simulink model "QPSK_send_new"  (Simulink 9.0)
settings: Solver=FixedStepDiscrete  StartTime=0.0  StopTime=inf  RelTol=1e-3
PreLoadFcn:
  | setenv('MW_MINGW64_LOC','C:\TDM-GCC-64')
  | load('qpsktxrx.mat')
StartFcn:
  | load('qpsktxrx.mat')
  | tic
StopFcn:
  | toc;
values from neighbouring files (symbols this model uses):
  data_send = [data_send frame]    [myimg_transfer.m]    (also in test_data.m = [data_send, head, data(i:i+20*9-1)]; test_data_v2.m = [data_send, frame])
  qpsktxrx =     [qpsktxrx.mat]
undefined symbols (not defined in the file or in its folder): CRC, gcbh, none, rcfiltgaincompat, videoinput
libraries: UN_HIL_Lib x2, commcrc2 x1, imaqlib x1, commutil2 x1, dspsigops x1, commsequence2 x1, commdigbbndpm3 x1, commfilt2 x1
Description:
  | QPSK Transmitter and Receiver.
  | 
  | This model shows the implementation of a QPSK transmitter and receiver.
settings Model: FPTRunName=Active  Creator=The MathWorks Inc.  LastModifiedBy=minel
settings DataIOCC: LimitDataPoints=on  SignalLoggingSaveFormat=ModelDataLogs  SaveOutput=off  SaveTime=off
settings OptimizationCC: BooleanDataType=off  DefaultParameterBehavior=Inlined  ExpressionDepthLimit=2147483647  LocalBlockOutputs=off
settings DebuggingCC: AlgebraicLoopMsg=error  SolverPrmCheckMsg=warning  SingleTaskRateTransMsg=error  ParameterPrecisionLossMsg=none  FcnCallInpInsideContextMsg=warning  StateNameClashWarn=warning
settings HardwareCC: TargetBitPerPointer=64  TargetBitPerSizeT=64  TargetBitPerPtrDiffT=64  TargetLongLongMode=on  TargetIntDivRoundTo=Zero  TargetEndianess=LittleEndian  TargetWordSize=64  TargetHWDeviceType=Generic->MATLAB Host Computer  ProdEqTarget=off
settings GRTTargetCC: GeneratePreprocessorConditionals=Disable all
settings ConfigComp: CovSFcnEnable=off
settings SimEventsCC: propDiagStatOutput=1  propPreventDuplicateEvents=0

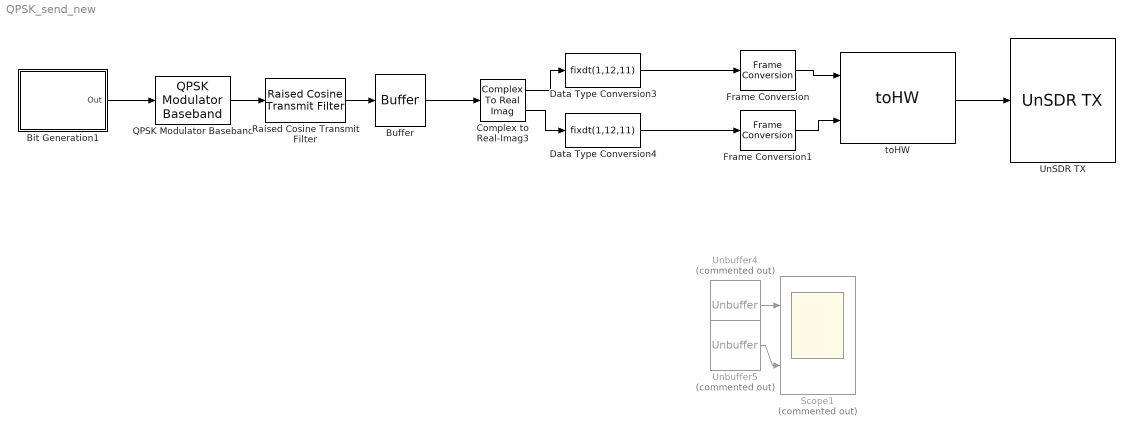
== system QPSK_send_new ==
  Bit Generation1 : Subsystem
      mask Display: disp('Bits Generation')
  Buffer : Buffer  N=4096  OutputFrames=off
  Complex to Real-Imag3 : ComplexToRealImag
  Data Type Conversion3 : DataTypeConversion  OutDataTypeStr=fixdt(1,12,11)
  Data Type Conversion4 : DataTypeConversion  OutDataTypeStr=fixdt(1,12,11)
  Frame Conversion : FrameConversion  InheritSamplingMode=off  OutFrame=Sample-based
  Frame Conversion1 : FrameConversion  InheritSamplingMode=off  OutFrame=Sample-based
  QPSK Modulator Baseband : commdigbbndpm3/QPSK Modulator Baseband  InType=Bit  Enc=Gray  Ph=pi/4  outDtype=double  outWordLen=16  outUDDataType=sfix(16)  outFracLenMode=Best precision  outFracLen=15  outDataTypeStr=double  outLastDataTypeStr=double
  Raised Cosine Transmit Filter : commfilt2/Raised Cosine Transmit Filter  filtType=Square root  R=0.5  filtSpan=2*((qpsktxrx.RaisedCosineFilterSpan)/2)  N=qpsktxrx.Upsampling  filterGain=rcfiltgaincompat(gcbh)  InputProcessing=Columns as channels (frame based)  RateOptions=Enforce single-rate processing  framing=Mute  checkCoeff=off  variableName=rcTxFilt  checkGain=Normalized  sampMode=Mute  saveAsFlag=0  currentFiltSpan=2*((qpsktxrx.RaisedCosineFilterSpan)/2)  D=(qpsktxrx.RaisedCosineFilterSpan)/2  launchFVT=off  roundingMode=Floor  overflowMode=off  coeffDataTypeStr=Inherit: Same word length as input  coeffMin=[]  coeffMax=[]  coeffLastDataTypeStr=Inherit: Same word length as input  outputDataTypeStr=Inherit: Same as accumulator  outputMin=[]  outputMax=[]  outputLastDataTypeStr=Inherit: Same as accumulator
  Scope1 : Scope  Commented=on  NumInputPorts=2
  UnSDR TX : UN_HIL_Lib/UnSDR TX  SystemSampleTime=-1
      settings: SourceProductName=HIL Blockset
  Unbuffer4 : Unbuffer  Commented=on
  Unbuffer5 : Unbuffer  Commented=on
  toHW : UN_HIL_Lib/toHW  SystemSampleTime=-1
      settings: SourceProductName=HIL Blockset
  wires:
  Unbuffer5/1 -> Scope1/2
  Unbuffer4/1 -> Scope1/1
  Data Type Conversion3/1 -> Frame Conversion/1
  Data Type Conversion4/1 -> Frame Conversion1/1
  Complex to Real-Imag3/2 -> Data Type Conversion4/1
  Complex to Real-Imag3/1 -> Data Type Conversion3/1
  Bit Generation1/1(Out) -> QPSK Modulator Baseband/1
  QPSK Modulator Baseband/1 -> Raised Cosine Transmit Filter/1
  toHW/1 -> UnSDR TX/1
  Frame Conversion/1 -> toHW/1
  Frame Conversion1/1 -> toHW/2
  Raised Cosine Transmit Filter/1 -> Buffer/1
  Buffer/1 -> Complex to Real-Imag3/1

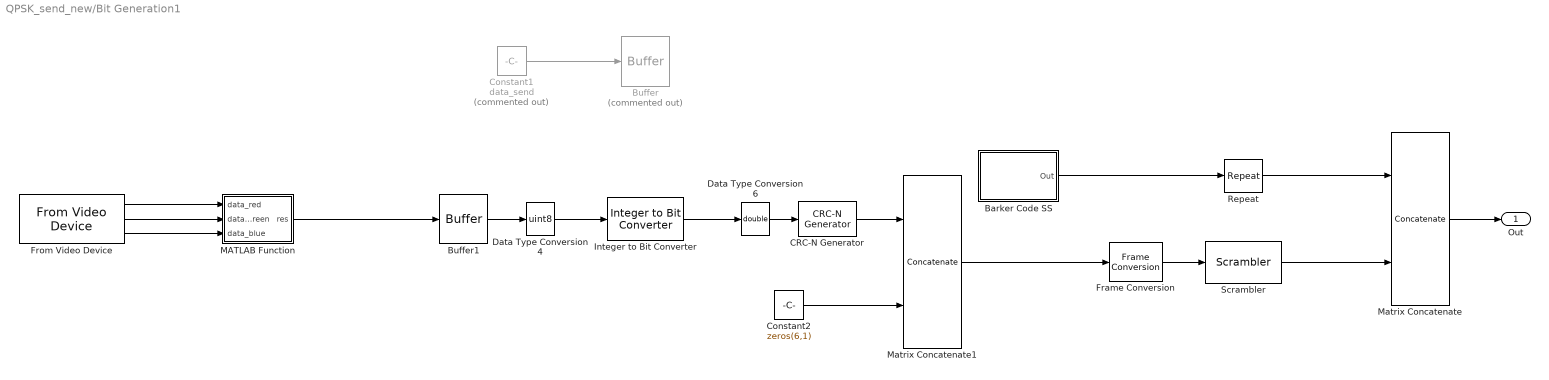
== system QPSK_send_new/Bit Generation1 ==
  Barker Code SS : Subsystem
      mask Display: disp('Unipolar\nBarker Code')
  Buffer : Buffer  Commented=on  N=20  OutputFrames=off
  Buffer1 : Buffer  N=20  OutputFrames=off
  CRC-N Generator : commcrc2/CRC-N Generator  crcMethod=CRC-8  iniStates=[0]  numChecksums=1
      settings: SourceProductName=Communications System Toolbox  SourceProductBaseCode=CM
  Constant1 : Constant  Commented=on  Value=data_send  SampleTime=1/2100/5*102470*5*5250*4096/1e8
  Constant2 : Constant  Value=zeros(6,1)  VectorParams1D=off  SampleTime=-1
  Data Type Conversion4 : DataTypeConversion  OutDataTypeStr=uint8
  Data Type Conversion6 : DataTypeConversion  OutDataTypeStr=double
  Frame Conversion : FrameConversion  InheritSamplingMode=off  OutFrame=Sample-based
  From Video Device : imaqlib/From Video Device  DeviceMenu=winvideo 1 (Integrated Webcam)  Device=winvideo 1 (Integrated Webcam)  ObjConstructor=videoinput('winvideo', 1)  VideoFormatMenu=YUY2_640x480  VideoFormat=YUY2_640x480  VideoSource=input1  ROIPosition=[0 0 480 640]  EnableHWTrigger=off  TriggerConfiguration=none/none  SampleTime=61620/1e4  OutputPortsMode=Separate color signals  DataType=uint8  CanDoHWTrigger=no  ReturnedColorSpace=rgb  BlockHandle=2351.0751  ROIWidth=640  ROIHeight=480  ROIColumn=0  ROIRow=0  EngXMLPath=D:\MATLAB2017\toolbox\imaq\imaq\private  DevXMLPath=C:\ProgramData\MATLAB\SupportPackages\R2017b\toolbox\imaq\supportpackages\genericvideo\adaptor\win64  EngLibPath=D:\MATLAB2017\toolbox\imaq\imaqblks\imaqmex\win64  ColorSpace=rgb  BayerSensorAlignment=grbg
      settings: SourceProductName=Image Acquisition Toolbox
  Integer to Bit Converter : commutil2/Integer to Bit Converter  nbits=8  signedInputValues=Unsigned  bitOrder=MSB first  outDtype=Inherit via internal rule
  MATLAB Function : MATLAB Function  TreatAsAtomicUnit=on
  Matrix Concatenate : Concatenate  Mode=Multidimensional array
  Matrix Concatenate1 : Concatenate  Mode=Multidimensional array
  Repeat : dspsigops/Repeat  N=2  InputProcessing=Columns as channels (frame based)  RateOptions=Enforce single-rate processing  ic=0  mode=Unused parameter value
      settings: SourceProductName=DSP System Toolbox
  Scrambler : commsequence2/Scrambler  M=2  poly=[1 1 1 0 1]  iniStaSource=Dialog Parameter  ini_sta=[0 0 0 0]  resetViaPort=off
      settings: SourceProductName=Communications System Toolbox  SourceProductBaseCode=CM
  Out : Outport
  wires:
  Constant2/1 -> Matrix Concatenate1/2
  Frame Conversion/1 -> Scrambler/1
  Scrambler/1 -> Matrix Concatenate/2
  Repeat/1 -> Matrix Concatenate/1
  Matrix Concatenate1/1 -> Frame Conversion/1
  Matrix Concatenate/1 -> Out/1
  Barker Code SS/1(Out) -> Repeat/1
  Integer to Bit Converter/1 -> Data Type Conversion6/1
  Data Type Conversion4/1 -> Integer to Bit Converter/1
  Data Type Conversion6/1 -> CRC-N Generator/1
  CRC-N Generator/1 -> Matrix Concatenate1/1
  From Video Device/3 -> MATLAB Function/3(data_blue)
  From Video Device/1 -> MATLAB Function/1(data_red)
  From Video Device/2 -> MATLAB Function/2(data_green)
  MATLAB Function/1(res) -> Buffer1/1
  Constant1/1 -> Buffer/1
  Buffer1/1 -> Data Type Conversion4/1

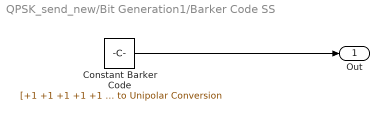
== system QPSK_send_new/Bit Generation1/Barker Code SS ==
  Constant Barker Code : Constant  Value=|  VectorParams1D=off  OutDataTypeStr=double  SampleTime=-1
      | [+1 +1 +1 +1 +1 -1 -1 +1 +1 -1 +1 -1 +1
      | ].' > 0  % Bipolar to Unipolar Conversion
  Out : Outport
  wires:
  Constant Barker Code/1 -> Out/1

== matlab function Bit Generation1/MATLAB Function ==
  data: data_red input double; res output double; data_green input double; data_blue input double
function res = img_transfer(data_red, data_green, data_blue)
    len = 61620;
    len2 = (len-180)/3;
    res = zeros(len,1);
    
%     [len_row,len_column] = size(data);
    len_row = 128;  
    len_column = 128;
    data_red=imresize(data_red,[len_row,len_column]);
    data_green=imresize(data_green,[len_row,len_column]);
    data_blue=imresize(data_blue,[len_row,len_column]);
    img = zeros(len_row,len_column,3);
    img(:,:,1) = uint8(data_red);
    img(:,:,2) = uint8(data_green);
    img(:,:,3) = uint8(data_blue);
    frame_size = 16;
    head_size = 4;
    %成帧
    %插入空帧，用于升余弦滤波器
    for img_num = 1:3
        data = data_transform(img(:,:,img_num), len_row, len_column);%128*128数据转为1维矩阵
        data = fixdata(data, frame_size);%补齐数组
        data_idx = 1;
        data_send = zeros(len2,1);
        for i = 1:frame_size:length(data)-frame_size
            row = ceil(i/len_column);
            column = i - len_column * (row-1);
            frame = [255, row, column, img_num, data(i:i+frame_size-1)];
            data_send(data_idx:data_idx+frame_size-1 + head_size) = frame';
            data_idx = data_idx + frame_size + head_size;
    %         data_send = [data_send;frame'];
        end
        res((img_num-1)*len2+181:img_num*len2+180) = data_send;
    end
end
